simulink model "section_6_2_second_group"  (R2020a)
settings: Solver=ode45  StartTime=0.0  StopTime=50  RelTol=1e-5  EnableMultiTasking=on
(part 4 of 4)

== matlab function section_6_2_second_group/FUZZY2/fuzzy_adaptive_law2 ==
  data: wdot output; x1 input; x2 input; x3 input; zz input; w input
function wdot   = fcn(x1,x2,x3,zz,w)
delta=0.01;
ux1=zeros(5,1);
ux2=zeros(5,1);
ux3=zeros(5,1);
%%x1 5条模糊规则

z=zeros(5,6);
for j=1:5
    z(j,1)=-2+j-delta;
end
for j=6:10
    z(j-5,2)=-2+(j-5)-delta;
end
for j=11:15
    z(j-10,3)=-2+(j-10)-delta;
end

h1=1;%%规则间距
if x1<=-2-delta
    ux1(1,1)=1;
end

if x1>=-2-delta&&x1<=-1-delta
    ux1(1,1)=0.5*sin(pi*(x1-(-2-delta))/h1+0.5*pi)+0.5;
end

if x1>=-2-delta&&x1<=0-delta
    ux1(2,1)=0.5*sin(pi*(x1-(-1-delta))/h1+0.5*pi)+0.5;
end

if x1>=-1-delta&&x1<=1-delta
    ux1(3,1)=0.5*sin(pi*(x1-(0-delta))/h1+0.5*pi)+0.5;
end

if x1>=0-delta&&x1<=2-delta
    ux1(4,1)=0.5*sin(pi*(x1-(1-delta))/h1+0.5*pi)+0.5;
end

if x1>=1-delta&&x1<=2-delta
    ux1(5,1)=0.5*sin(pi*(x1-(2-delta))/h1+0.5*pi)+0.5;
end

if x1>2-delta
    ux1(5,1)=1;
end


h2=1;%%规则间距
if x2<=-2-delta
    ux2(1,1)=1;
end

if x2>=-2-delta&&x2<=-1-delta
    ux2(1,1)=0.5*sin(pi*(x2-(-2-delta))/h2+0.5*pi)+0.5;
end

if x2>=-2-delta&&x2<=0-delta
    ux2(2,1)=0.5*sin(pi*(x2-(-1-delta))/h2+0.5*pi)+0.5;
end

if x2>=-1-delta&&x2<=1-delta
    ux2(3,1)=0.5*sin(pi*(x2-(0-delta))/h2+0.5*pi)+0.5;
end

if x2>=0-delta&&x2<=2-delta
    ux2(4,1)=0.5*sin(pi*(x2-(1-delta))/h2+0.5*pi)+0.5;
end

if x2>=1-delta&&x2<=2-delta
    ux2(5,1)=0.5*sin(pi*(x2-(2-delta))/h2+0.5*pi)+0.5;
end

if x2>2-delta
    ux2(5,1)=1;
end

h3=1;%%规则间距
if x3<=-2-delta
    ux3(1,1)=1;
end

if x3>=-2-delta&&x3<=-1-delta
    ux3(1,1)=0.5*sin(pi*(x3-(-2-delta))/h3+0.5*pi)+0.5;
end

if x3>=-2-delta&&x3<=0-delta
    ux3(2,1)=0.5*sin(pi*(x3-(-1-delta))/h3+0.5*pi)+0.5;
end

if x3>=-1-delta&&x3<=1-delta
    ux3(3,1)=0.5*sin(pi*(x3-(0-delta))/h3+0.5*pi)+0.5;
end

if x3>=0-delta&&x3<=2-delta
    ux3(4,1)=0.5*sin(pi*(x3-(1-delta))/h3+0.5*pi)+0.5;
end

if x3>=1-delta&&x3<=2-delta
    ux3(5,1)=0.5*sin(pi*(x3-(2-delta))/h3+0.5*pi)+0.5;
end

if x3>2-delta
    ux3(5,1)=1;
end


%中心平均解模糊
Basic=0;
for i1=1:5
    for i2=1:5
        for i3=1:5
            Basic=Basic+ux1(i1,1)*ux2(i2,1)*ux3(i3,1);  
        end
    end
end

beta=zeros(5,5,5);
for i1=1:5
    for i2=1:5
        for i3=1:5
            beta(i1,i2,i3)=ux1(i1,1)*ux2(i2,1)*ux3(i3,1)/Basic;
        end
    end
end

wdot=zeros(5,5,5);
for i1=1:5
    for i2=1:5
        for i3=1:5
            wdot(i1,i2,i3)=w*beta(i1,i2,i3)*zz*z(i3,1);
        end
    end
end

end

== matlab function section_6_2_second_group/FUZZY2/fuzzy_adaptive_law3 ==
  data: wdot output; x1 input; x2 input; x3 input; zz input; w input
function wdot   = fcn(x1,x2,x3,zz,w)
delta=0.01;
ux1=zeros(5,1);
ux2=zeros(5,1);
ux3=zeros(5,1);
%%x1 5条模糊规则

z=zeros(5,6);
for j=1:5
    z(j,1)=-2+j-delta;
end
for j=6:10
    z(j-5,2)=-2+(j-5)-delta;
end
for j=11:15
    z(j-10,3)=-2+(j-10)-delta;
end

h1=1;%%规则间距
if x1<=-2-delta
    ux1(1,1)=1;
end

if x1>=-2-delta&&x1<=-1-delta
    ux1(1,1)=0.5*sin(pi*(x1-(-2-delta))/h1+0.5*pi)+0.5;
end

if x1>=-2-delta&&x1<=0-delta
    ux1(2,1)=0.5*sin(pi*(x1-(-1-delta))/h1+0.5*pi)+0.5;
end

if x1>=-1-delta&&x1<=1-delta
    ux1(3,1)=0.5*sin(pi*(x1-(0-delta))/h1+0.5*pi)+0.5;
end

if x1>=0-delta&&x1<=2-delta
    ux1(4,1)=0.5*sin(pi*(x1-(1-delta))/h1+0.5*pi)+0.5;
end

if x1>=1-delta&&x1<=2-delta
    ux1(5,1)=0.5*sin(pi*(x1-(2-delta))/h1+0.5*pi)+0.5;
end

if x1>2-delta
    ux1(5,1)=1;
end


h2=1;%%规则间距
if x2<=-2-delta
    ux2(1,1)=1;
end

if x2>=-2-delta&&x2<=-1-delta
    ux2(1,1)=0.5*sin(pi*(x2-(-2-delta))/h2+0.5*pi)+0.5;
end

if x2>=-2-delta&&x2<=0-delta
    ux2(2,1)=0.5*sin(pi*(x2-(-1-delta))/h2+0.5*pi)+0.5;
end

if x2>=-1-delta&&x2<=1-delta
    ux2(3,1)=0.5*sin(pi*(x2-(0-delta))/h2+0.5*pi)+0.5;
end

if x2>=0-delta&&x2<=2-delta
    ux2(4,1)=0.5*sin(pi*(x2-(1-delta))/h2+0.5*pi)+0.5;
end

if x2>=1-delta&&x2<=2-delta
    ux2(5,1)=0.5*sin(pi*(x2-(2-delta))/h2+0.5*pi)+0.5;
end

if x2>2-delta
    ux2(5,1)=1;
end

h3=1;%%规则间距
if x3<=-2-delta
    ux3(1,1)=1;
end

if x3>=-2-delta&&x3<=-1-delta
    ux3(1,1)=0.5*sin(pi*(x3-(-2-delta))/h3+0.5*pi)+0.5;
end

if x3>=-2-delta&&x3<=0-delta
    ux3(2,1)=0.5*sin(pi*(x3-(-1-delta))/h3+0.5*pi)+0.5;
end

if x3>=-1-delta&&x3<=1-delta
    ux3(3,1)=0.5*sin(pi*(x3-(0-delta))/h3+0.5*pi)+0.5;
end

if x3>=0-delta&&x3<=2-delta
    ux3(4,1)=0.5*sin(pi*(x3-(1-delta))/h3+0.5*pi)+0.5;
end

if x3>=1-delta&&x3<=2-delta
    ux3(5,1)=0.5*sin(pi*(x3-(2-delta))/h3+0.5*pi)+0.5;
end

if x3>2-delta
    ux3(5,1)=1;
end


%中心平均解模糊
Basic=0;
for i1=1:5
    for i2=1:5
        for i3=1:5
            Basic=Basic+ux1(i1,1)*ux2(i2,1)*ux3(i3,1);  
        end
    end
end

beta=zeros(5,5,5);
for i1=1:5
    for i2=1:5
        for i3=1:5
            beta(i1,i2,i3)=ux1(i1,1)*ux2(i2,1)*ux3(i3,1)/Basic;
        end
    end
end

wdot=zeros(5,5,5);
for i1=1:5
    for i2=1:5
        for i3=1:5
            wdot(i1,i2,i3)=w*beta(i1,i2,i3)*zz*z(i3,1);
        end
    end
end

end

== matlab function section_6_2_second_group/FUZZY2/fuzzy_adaptive_law4 ==
  data: wdot output; x1 input; x2 input; x3 input; zz input; w input
function wdot   = fcn(x1,x2,x3,zz,w)
delta=0.01;
ux1=zeros(5,1);
ux2=zeros(5,1);
ux3=zeros(5,1);
%%x1 5条模糊规则

z=zeros(5,6);
for j=1:5
    z(j,1)=-2+j-delta;
end
for j=6:10
    z(j-5,2)=-2+(j-5)-delta;
end
for j=11:15
    z(j-10,3)=-2+(j-10)-delta;
end

h1=1;%%规则间距
if x1<=-2-delta
    ux1(1,1)=1;
end

if x1>=-2-delta&&x1<=-1-delta
    ux1(1,1)=0.5*sin(pi*(x1-(-2-delta))/h1+0.5*pi)+0.5;
end

if x1>=-2-delta&&x1<=0-delta
    ux1(2,1)=0.5*sin(pi*(x1-(-1-delta))/h1+0.5*pi)+0.5;
end

if x1>=-1-delta&&x1<=1-delta
    ux1(3,1)=0.5*sin(pi*(x1-(0-delta))/h1+0.5*pi)+0.5;
end

if x1>=0-delta&&x1<=2-delta
    ux1(4,1)=0.5*sin(pi*(x1-(1-delta))/h1+0.5*pi)+0.5;
end

if x1>=1-delta&&x1<=2-delta
    ux1(5,1)=0.5*sin(pi*(x1-(2-delta))/h1+0.5*pi)+0.5;
end

if x1>2-delta
    ux1(5,1)=1;
end


h2=1;%%规则间距
if x2<=-2-delta
    ux2(1,1)=1;
end

if x2>=-2-delta&&x2<=-1-delta
    ux2(1,1)=0.5*sin(pi*(x2-(-2-delta))/h2+0.5*pi)+0.5;
end

if x2>=-2-delta&&x2<=0-delta
    ux2(2,1)=0.5*sin(pi*(x2-(-1-delta))/h2+0.5*pi)+0.5;
end

if x2>=-1-delta&&x2<=1-delta
    ux2(3,1)=0.5*sin(pi*(x2-(0-delta))/h2+0.5*pi)+0.5;
end

if x2>=0-delta&&x2<=2-delta
    ux2(4,1)=0.5*sin(pi*(x2-(1-delta))/h2+0.5*pi)+0.5;
end

if x2>=1-delta&&x2<=2-delta
    ux2(5,1)=0.5*sin(pi*(x2-(2-delta))/h2+0.5*pi)+0.5;
end

if x2>2-delta
    ux2(5,1)=1;
end

h3=1;%%规则间距
if x3<=-2-delta
    ux3(1,1)=1;
end

if x3>=-2-delta&&x3<=-1-delta
    ux3(1,1)=0.5*sin(pi*(x3-(-2-delta))/h3+0.5*pi)+0.5;
end

if x3>=-2-delta&&x3<=0-delta
    ux3(2,1)=0.5*sin(pi*(x3-(-1-delta))/h3+0.5*pi)+0.5;
end

if x3>=-1-delta&&x3<=1-delta
    ux3(3,1)=0.5*sin(pi*(x3-(0-delta))/h3+0.5*pi)+0.5;
end

if x3>=0-delta&&x3<=2-delta
    ux3(4,1)=0.5*sin(pi*(x3-(1-delta))/h3+0.5*pi)+0.5;
end

if x3>=1-delta&&x3<=2-delta
    ux3(5,1)=0.5*sin(pi*(x3-(2-delta))/h3+0.5*pi)+0.5;
end

if x3>2-delta
    ux3(5,1)=1;
end


%中心平均解模糊
Basic=0;
for i1=1:5
    for i2=1:5
        for i3=1:5
            Basic=Basic+ux1(i1,1)*ux2(i2,1)*ux3(i3,1);  
        end
    end
end

beta=zeros(5,5,5);
for i1=1:5
    for i2=1:5
        for i3=1:5
            beta(i1,i2,i3)=ux1(i1,1)*ux2(i2,1)*ux3(i3,1)/Basic;
        end
    end
end

wdot=zeros(5,5,5);
for i1=1:5
    for i2=1:5
        for i3=1:5
            wdot(i1,i2,i3)=w*beta(i1,i2,i3)*zz*z(i3,1);
        end
    end
end

end

== matlab function section_6_2_second_group/FUZZY2/fuzzy_adaptive_law5 ==
  data: wdot output; x1 input; x2 input; x3 input; zz input; w input
function wdot   = fcn(x1,x2,x3,zz,w)
delta=0.01;
ux1=zeros(5,1);
ux2=zeros(5,1);
ux3=zeros(5,1);
%%x1 5条模糊规则

z=zeros(5,6);
for j=1:5
    z(j,1)=-2+j-delta;
end
for j=6:10
    z(j-5,2)=-2+(j-5)-delta;
end
for j=11:15
    z(j-10,3)=-2+(j-10)-delta;
end

h1=1;%%规则间距
if x1<=-2-delta
    ux1(1,1)=1;
end

if x1>=-2-delta&&x1<=-1-delta
    ux1(1,1)=0.5*sin(pi*(x1-(-2-delta))/h1+0.5*pi)+0.5;
end

if x1>=-2-delta&&x1<=0-delta
    ux1(2,1)=0.5*sin(pi*(x1-(-1-delta))/h1+0.5*pi)+0.5;
end

if x1>=-1-delta&&x1<=1-delta
    ux1(3,1)=0.5*sin(pi*(x1-(0-delta))/h1+0.5*pi)+0.5;
end

if x1>=0-delta&&x1<=2-delta
    ux1(4,1)=0.5*sin(pi*(x1-(1-delta))/h1+0.5*pi)+0.5;
end

if x1>=1-delta&&x1<=2-delta
    ux1(5,1)=0.5*sin(pi*(x1-(2-delta))/h1+0.5*pi)+0.5;
end

if x1>2-delta
    ux1(5,1)=1;
end


h2=1;%%规则间距
if x2<=-2-delta
    ux2(1,1)=1;
end

if x2>=-2-delta&&x2<=-1-delta
    ux2(1,1)=0.5*sin(pi*(x2-(-2-delta))/h2+0.5*pi)+0.5;
end

if x2>=-2-delta&&x2<=0-delta
    ux2(2,1)=0.5*sin(pi*(x2-(-1-delta))/h2+0.5*pi)+0.5;
end

if x2>=-1-delta&&x2<=1-delta
    ux2(3,1)=0.5*sin(pi*(x2-(0-delta))/h2+0.5*pi)+0.5;
end

if x2>=0-delta&&x2<=2-delta
    ux2(4,1)=0.5*sin(pi*(x2-(1-delta))/h2+0.5*pi)+0.5;
end

if x2>=1-delta&&x2<=2-delta
    ux2(5,1)=0.5*sin(pi*(x2-(2-delta))/h2+0.5*pi)+0.5;
end

if x2>2-delta
    ux2(5,1)=1;
end

h3=1;%%规则间距
if x3<=-2-delta
    ux3(1,1)=1;
end

if x3>=-2-delta&&x3<=-1-delta
    ux3(1,1)=0.5*sin(pi*(x3-(-2-delta))/h3+0.5*pi)+0.5;
end

if x3>=-2-delta&&x3<=0-delta
    ux3(2,1)=0.5*sin(pi*(x3-(-1-delta))/h3+0.5*pi)+0.5;
end

if x3>=-1-delta&&x3<=1-delta
    ux3(3,1)=0.5*sin(pi*(x3-(0-delta))/h3+0.5*pi)+0.5;
end

if x3>=0-delta&&x3<=2-delta
    ux3(4,1)=0.5*sin(pi*(x3-(1-delta))/h3+0.5*pi)+0.5;
end

if x3>=1-delta&&x3<=2-delta
    ux3(5,1)=0.5*sin(pi*(x3-(2-delta))/h3+0.5*pi)+0.5;
end

if x3>2-delta
    ux3(5,1)=1;
end


%中心平均解模糊
Basic=0;
for i1=1:5
    for i2=1:5
        for i3=1:5
            Basic=Basic+ux1(i1,1)*ux2(i2,1)*ux3(i3,1);  
        end
    end
end

beta=zeros(5,5,5);
for i1=1:5
    for i2=1:5
        for i3=1:5
            beta(i1,i2,i3)=ux1(i1,1)*ux2(i2,1)*ux3(i3,1)/Basic;
        end
    end
end

wdot=zeros(5,5,5);
for i1=1:5
    for i2=1:5
        for i3=1:5
            wdot(i1,i2,i3)=w*beta(i1,i2,i3)*zz*z(i3,1);
        end
    end
end

end

== matlab function section_6_2_second_group/FUZZY2/fuzzy_adaptive_law6 ==
  data: wdot output; x1 input; x2 input; x3 input; zz input; w input
function wdot   = fcn(x1,x2,x3,zz,w)
delta=0.01;
ux1=zeros(5,1);
ux2=zeros(5,1);
ux3=zeros(5,1);
%%x1 5条模糊规则

z=zeros(5,6);
for j=1:5
    z(j,1)=-2+j-delta;
end
for j=6:10
    z(j-5,2)=-2+(j-5)-delta;
end
for j=11:15
    z(j-10,3)=-2+(j-10)-delta;
end

h1=1;%%规则间距
if x1<=-2-delta
    ux1(1,1)=1;
end

if x1>=-2-delta&&x1<=-1-delta
    ux1(1,1)=0.5*sin(pi*(x1-(-2-delta))/h1+0.5*pi)+0.5;
end

if x1>=-2-delta&&x1<=0-delta
    ux1(2,1)=0.5*sin(pi*(x1-(-1-delta))/h1+0.5*pi)+0.5;
end

if x1>=-1-delta&&x1<=1-delta
    ux1(3,1)=0.5*sin(pi*(x1-(0-delta))/h1+0.5*pi)+0.5;
end

if x1>=0-delta&&x1<=2-delta
    ux1(4,1)=0.5*sin(pi*(x1-(1-delta))/h1+0.5*pi)+0.5;
end

if x1>=1-delta&&x1<=2-delta
    ux1(5,1)=0.5*sin(pi*(x1-(2-delta))/h1+0.5*pi)+0.5;
end

if x1>2-delta
    ux1(5,1)=1;
end


h2=1;%%规则间距
if x2<=-2-delta
    ux2(1,1)=1;
end

if x2>=-2-delta&&x2<=-1-delta
    ux2(1,1)=0.5*sin(pi*(x2-(-2-delta))/h2+0.5*pi)+0.5;
end

if x2>=-2-delta&&x2<=0-delta
    ux2(2,1)=0.5*sin(pi*(x2-(-1-delta))/h2+0.5*pi)+0.5;
end

if x2>=-1-delta&&x2<=1-delta
    ux2(3,1)=0.5*sin(pi*(x2-(0-delta))/h2+0.5*pi)+0.5;
end

if x2>=0-delta&&x2<=2-delta
    ux2(4,1)=0.5*sin(pi*(x2-(1-delta))/h2+0.5*pi)+0.5;
end

if x2>=1-delta&&x2<=2-delta
    ux2(5,1)=0.5*sin(pi*(x2-(2-delta))/h2+0.5*pi)+0.5;
end

if x2>2-delta
    ux2(5,1)=1;
end

h3=1;%%规则间距
if x3<=-2-delta
    ux3(1,1)=1;
end

if x3>=-2-delta&&x3<=-1-delta
    ux3(1,1)=0.5*sin(pi*(x3-(-2-delta))/h3+0.5*pi)+0.5;
end

if x3>=-2-delta&&x3<=0-delta
    ux3(2,1)=0.5*sin(pi*(x3-(-1-delta))/h3+0.5*pi)+0.5;
end

if x3>=-1-delta&&x3<=1-delta
    ux3(3,1)=0.5*sin(pi*(x3-(0-delta))/h3+0.5*pi)+0.5;
end

if x3>=0-delta&&x3<=2-delta
    ux3(4,1)=0.5*sin(pi*(x3-(1-delta))/h3+0.5*pi)+0.5;
end

if x3>=1-delta&&x3<=2-delta
    ux3(5,1)=0.5*sin(pi*(x3-(2-delta))/h3+0.5*pi)+0.5;
end

if x3>2-delta
    ux3(5,1)=1;
end


%中心平均解模糊
Basic=0;
for i1=1:5
    for i2=1:5
        for i3=1:5
            Basic=Basic+ux1(i1,1)*ux2(i2,1)*ux3(i3,1);  
        end
    end
end

beta=zeros(5,5,5);
for i1=1:5
    for i2=1:5
        for i3=1:5
            beta(i1,i2,i3)=ux1(i1,1)*ux2(i2,1)*ux3(i3,1)/Basic;
        end
    end
end

wdot=zeros(5,5,5);
for i1=1:5
    for i2=1:5
        for i3=1:5
            wdot(i1,i2,i3)=w*beta(i1,i2,i3)*zz*z(i3,1);
        end
    end
end

end

== matlab function section_6_2_second_group/FUZZY2/fuzzy_adaptive_law7 ==
  data: wdot output; x1 input; x2 input; x3 input; zz input; w input
function wdot   = fcn(x1,x2,x3,zz,w)
delta=0.01;
ux1=zeros(5,1);
ux2=zeros(5,1);
ux3=zeros(5,1);
%%x1 5条模糊规则

z=zeros(5,6);
for j=1:5
    z(j,1)=-2+j-delta;
end
for j=6:10
    z(j-5,2)=-2+(j-5)-delta;
end
for j=11:15
    z(j-10,3)=-2+(j-10)-delta;
end

h1=1;%%规则间距
if x1<=-2-delta
    ux1(1,1)=1;
end

if x1>=-2-delta&&x1<=-1-delta
    ux1(1,1)=0.5*sin(pi*(x1-(-2-delta))/h1+0.5*pi)+0.5;
end

if x1>=-2-delta&&x1<=0-delta
    ux1(2,1)=0.5*sin(pi*(x1-(-1-delta))/h1+0.5*pi)+0.5;
end

if x1>=-1-delta&&x1<=1-delta
    ux1(3,1)=0.5*sin(pi*(x1-(0-delta))/h1+0.5*pi)+0.5;
end

if x1>=0-delta&&x1<=2-delta
    ux1(4,1)=0.5*sin(pi*(x1-(1-delta))/h1+0.5*pi)+0.5;
end

if x1>=1-delta&&x1<=2-delta
    ux1(5,1)=0.5*sin(pi*(x1-(2-delta))/h1+0.5*pi)+0.5;
end

if x1>2-delta
    ux1(5,1)=1;
end


h2=1;%%规则间距
if x2<=-2-delta
    ux2(1,1)=1;
end

if x2>=-2-delta&&x2<=-1-delta
    ux2(1,1)=0.5*sin(pi*(x2-(-2-delta))/h2+0.5*pi)+0.5;
end

if x2>=-2-delta&&x2<=0-delta
    ux2(2,1)=0.5*sin(pi*(x2-(-1-delta))/h2+0.5*pi)+0.5;
end

if x2>=-1-delta&&x2<=1-delta
    ux2(3,1)=0.5*sin(pi*(x2-(0-delta))/h2+0.5*pi)+0.5;
end

if x2>=0-delta&&x2<=2-delta
    ux2(4,1)=0.5*sin(pi*(x2-(1-delta))/h2+0.5*pi)+0.5;
end

if x2>=1-delta&&x2<=2-delta
    ux2(5,1)=0.5*sin(pi*(x2-(2-delta))/h2+0.5*pi)+0.5;
end

if x2>2-delta
    ux2(5,1)=1;
end

h3=1;%%规则间距
if x3<=-2-delta
    ux3(1,1)=1;
end

if x3>=-2-delta&&x3<=-1-delta
    ux3(1,1)=0.5*sin(pi*(x3-(-2-delta))/h3+0.5*pi)+0.5;
end

if x3>=-2-delta&&x3<=0-delta
    ux3(2,1)=0.5*sin(pi*(x3-(-1-delta))/h3+0.5*pi)+0.5;
end

if x3>=-1-delta&&x3<=1-delta
    ux3(3,1)=0.5*sin(pi*(x3-(0-delta))/h3+0.5*pi)+0.5;
end

if x3>=0-delta&&x3<=2-delta
    ux3(4,1)=0.5*sin(pi*(x3-(1-delta))/h3+0.5*pi)+0.5;
end

if x3>=1-delta&&x3<=2-delta
    ux3(5,1)=0.5*sin(pi*(x3-(2-delta))/h3+0.5*pi)+0.5;
end

if x3>2-delta
    ux3(5,1)=1;
end


%中心平均解模糊
Basic=0;
for i1=1:5
    for i2=1:5
        for i3=1:5
            Basic=Basic+ux1(i1,1)*ux2(i2,1)*ux3(i3,1);  
        end
    end
end

beta=zeros(5,5,5);
for i1=1:5
    for i2=1:5
        for i3=1:5
            beta(i1,i2,i3)=ux1(i1,1)*ux2(i2,1)*ux3(i3,1)/Basic;
        end
    end
end

wdot=zeros(5,5,5);
for i1=1:5
    for i2=1:5
        for i3=1:5
            wdot(i1,i2,i3)=w*beta(i1,i2,i3)*zz*z(i3,1);
        end
    end
end

end

== matlab function section_6_2_second_group/FUZZY2/fuzzy_adaptive_law8 ==
  data: wdot output; x1 input; x2 input; x3 input; zz input; w input
function wdot   = fcn(x1,x2,x3,zz,w)
delta=0.01;
ux1=zeros(5,1);
ux2=zeros(5,1);
ux3=zeros(5,1);
%%x1 5条模糊规则

z=zeros(5,6);
for j=1:5
    z(j,1)=-2+j-delta;
end
for j=6:10
    z(j-5,2)=-2+(j-5)-delta;
end
for j=11:15
    z(j-10,3)=-2+(j-10)-delta;
end

h1=1;%%规则间距
if x1<=-2-delta
    ux1(1,1)=1;
end

if x1>=-2-delta&&x1<=-1-delta
    ux1(1,1)=0.5*sin(pi*(x1-(-2-delta))/h1+0.5*pi)+0.5;
end

if x1>=-2-delta&&x1<=0-delta
    ux1(2,1)=0.5*sin(pi*(x1-(-1-delta))/h1+0.5*pi)+0.5;
end

if x1>=-1-delta&&x1<=1-delta
    ux1(3,1)=0.5*sin(pi*(x1-(0-delta))/h1+0.5*pi)+0.5;
end

if x1>=0-delta&&x1<=2-delta
    ux1(4,1)=0.5*sin(pi*(x1-(1-delta))/h1+0.5*pi)+0.5;
end

if x1>=1-delta&&x1<=2-delta
    ux1(5,1)=0.5*sin(pi*(x1-(2-delta))/h1+0.5*pi)+0.5;
end

if x1>2-delta
    ux1(5,1)=1;
end


h2=1;%%规则间距
if x2<=-2-delta
    ux2(1,1)=1;
end

if x2>=-2-delta&&x2<=-1-delta
    ux2(1,1)=0.5*sin(pi*(x2-(-2-delta))/h2+0.5*pi)+0.5;
end

if x2>=-2-delta&&x2<=0-delta
    ux2(2,1)=0.5*sin(pi*(x2-(-1-delta))/h2+0.5*pi)+0.5;
end

if x2>=-1-delta&&x2<=1-delta
    ux2(3,1)=0.5*sin(pi*(x2-(0-delta))/h2+0.5*pi)+0.5;
end

if x2>=0-delta&&x2<=2-delta
    ux2(4,1)=0.5*sin(pi*(x2-(1-delta))/h2+0.5*pi)+0.5;
end

if x2>=1-delta&&x2<=2-delta
    ux2(5,1)=0.5*sin(pi*(x2-(2-delta))/h2+0.5*pi)+0.5;
end

if x2>2-delta
    ux2(5,1)=1;
end

h3=1;%%规则间距
if x3<=-2-delta
    ux3(1,1)=1;
end

if x3>=-2-delta&&x3<=-1-delta
    ux3(1,1)=0.5*sin(pi*(x3-(-2-delta))/h3+0.5*pi)+0.5;
end

if x3>=-2-delta&&x3<=0-delta
    ux3(2,1)=0.5*sin(pi*(x3-(-1-delta))/h3+0.5*pi)+0.5;
end

if x3>=-1-delta&&x3<=1-delta
    ux3(3,1)=0.5*sin(pi*(x3-(0-delta))/h3+0.5*pi)+0.5;
end

if x3>=0-delta&&x3<=2-delta
    ux3(4,1)=0.5*sin(pi*(x3-(1-delta))/h3+0.5*pi)+0.5;
end

if x3>=1-delta&&x3<=2-delta
    ux3(5,1)=0.5*sin(pi*(x3-(2-delta))/h3+0.5*pi)+0.5;
end

if x3>2-delta
    ux3(5,1)=1;
end


%中心平均解模糊
Basic=0;
for i1=1:5
    for i2=1:5
        for i3=1:5
            Basic=Basic+ux1(i1,1)*ux2(i2,1)*ux3(i3,1);  
        end
    end
end

beta=zeros(5,5,5);
for i1=1:5
    for i2=1:5
        for i3=1:5
            beta(i1,i2,i3)=ux1(i1,1)*ux2(i2,1)*ux3(i3,1)/Basic;
        end
    end
end

wdot=zeros(5,5,5);
for i1=1:5
    for i2=1:5
        for i3=1:5
            wdot(i1,i2,i3)=w*beta(i1,i2,i3)*zz*z(i3,1);
        end
    end
end

end

== matlab function section_6_2_second_group/FUZZY2/fuzzy_adaptive_law9 ==
  data: wdot output; x1 input; x2 input; x3 input; zz input; w input
function wdot   = fcn(x1,x2,x3,zz,w)
delta=0.01;
ux1=zeros(5,1);
ux2=zeros(5,1);
ux3=zeros(5,1);
%%x1 5条模糊规则

z=zeros(5,6);
for j=1:5
    z(j,1)=-2+j-delta;
end
for j=6:10
    z(j-5,2)=-2+(j-5)-delta;
end
for j=11:15
    z(j-10,3)=-2+(j-10)-delta;
end

h1=1;%%规则间距
if x1<=-2-delta
    ux1(1,1)=1;
end

if x1>=-2-delta&&x1<=-1-delta
    ux1(1,1)=0.5*sin(pi*(x1-(-2-delta))/h1+0.5*pi)+0.5;
end

if x1>=-2-delta&&x1<=0-delta
    ux1(2,1)=0.5*sin(pi*(x1-(-1-delta))/h1+0.5*pi)+0.5;
end

if x1>=-1-delta&&x1<=1-delta
    ux1(3,1)=0.5*sin(pi*(x1-(0-delta))/h1+0.5*pi)+0.5;
end

if x1>=0-delta&&x1<=2-delta
    ux1(4,1)=0.5*sin(pi*(x1-(1-delta))/h1+0.5*pi)+0.5;
end

if x1>=1-delta&&x1<=2-delta
    ux1(5,1)=0.5*sin(pi*(x1-(2-delta))/h1+0.5*pi)+0.5;
end

if x1>2-delta
    ux1(5,1)=1;
end


h2=1;%%规则间距
if x2<=-2-delta
    ux2(1,1)=1;
end

if x2>=-2-delta&&x2<=-1-delta
    ux2(1,1)=0.5*sin(pi*(x2-(-2-delta))/h2+0.5*pi)+0.5;
end

if x2>=-2-delta&&x2<=0-delta
    ux2(2,1)=0.5*sin(pi*(x2-(-1-delta))/h2+0.5*pi)+0.5;
end

if x2>=-1-delta&&x2<=1-delta
    ux2(3,1)=0.5*sin(pi*(x2-(0-delta))/h2+0.5*pi)+0.5;
end

if x2>=0-delta&&x2<=2-delta
    ux2(4,1)=0.5*sin(pi*(x2-(1-delta))/h2+0.5*pi)+0.5;
end

if x2>=1-delta&&x2<=2-delta
    ux2(5,1)=0.5*sin(pi*(x2-(2-delta))/h2+0.5*pi)+0.5;
end

if x2>2-delta
    ux2(5,1)=1;
end

h3=1;%%规则间距
if x3<=-2-delta
    ux3(1,1)=1;
end

if x3>=-2-delta&&x3<=-1-delta
    ux3(1,1)=0.5*sin(pi*(x3-(-2-delta))/h3+0.5*pi)+0.5;
end

if x3>=-2-delta&&x3<=0-delta
    ux3(2,1)=0.5*sin(pi*(x3-(-1-delta))/h3+0.5*pi)+0.5;
end

if x3>=-1-delta&&x3<=1-delta
    ux3(3,1)=0.5*sin(pi*(x3-(0-delta))/h3+0.5*pi)+0.5;
end

if x3>=0-delta&&x3<=2-delta
    ux3(4,1)=0.5*sin(pi*(x3-(1-delta))/h3+0.5*pi)+0.5;
end

if x3>=1-delta&&x3<=2-delta
    ux3(5,1)=0.5*sin(pi*(x3-(2-delta))/h3+0.5*pi)+0.5;
end

if x3>2-delta
    ux3(5,1)=1;
end


%中心平均解模糊
Basic=0;
for i1=1:5
    for i2=1:5
        for i3=1:5
            Basic=Basic+ux1(i1,1)*ux2(i2,1)*ux3(i3,1);  
        end
    end
end

beta=zeros(5,5,5);
for i1=1:5
    for i2=1:5
        for i3=1:5
            beta(i1,i2,i3)=ux1(i1,1)*ux2(i2,1)*ux3(i3,1)/Basic;
        end
    end
end

wdot=zeros(5,5,5);
for i1=1:5
    for i2=1:5
        for i3=1:5
            wdot(i1,i2,i3)=w*beta(i1,i2,i3)*zz*z(i3,1);
        end
    end
end

end

== matlab function section_6_2_second_group/FUZZY2/fuzzy_logic_system1 ==
  data: aF output; x1 input; x2 input; x3 input; w input
function aF    = fcn(x1,x2,x3,w)
%%x1 5条模糊规则
delta=0.01;
ux1=zeros(5,1);
ux2=zeros(5,1);
ux3=zeros(5,1);
%%x1 5条模糊规则

h1=1;%%规则间距
if x1<=-2-delta
    ux1(1,1)=1;
end

if x1>=-2-delta&&x1<=-1-delta
    ux1(1,1)=0.5*sin(pi*(x1-(-2-delta))/h1+0.5*pi)+0.5;
end

if x1>=-2-delta&&x1<=0-delta
    ux1(2,1)=0.5*sin(pi*(x1-(-1-delta))/h1+0.5*pi)+0.5;
end

if x1>=-1-delta&&x1<=1-delta
    ux1(3,1)=0.5*sin(pi*(x1-(0-delta))/h1+0.5*pi)+0.5;
end

if x1>=0-delta&&x1<=2-delta
    ux1(4,1)=0.5*sin(pi*(x1-(1-delta))/h1+0.5*pi)+0.5;
end

if x1>=1-delta&&x1<=2-delta
    ux1(5,1)=0.5*sin(pi*(x1-(2-delta))/h1+0.5*pi)+0.5;
end

if x1>2-delta
    ux1(5,1)=1;
end


h2=1;%%规则间距
if x2<=-2-delta
    ux2(1,1)=1;
end

if x2>=-2-delta&&x2<=-1-delta
    ux2(1,1)=0.5*sin(pi*(x2-(-2-delta))/h2+0.5*pi)+0.5;
end

if x2>=-2-delta&&x2<=0-delta
    ux2(2,1)=0.5*sin(pi*(x2-(-1-delta))/h2+0.5*pi)+0.5;
end

if x2>=-1-delta&&x2<=1-delta
    ux2(3,1)=0.5*sin(pi*(x2-(0-delta))/h2+0.5*pi)+0.5;
end

if x2>=0-delta&&x2<=2-delta
    ux2(4,1)=0.5*sin(pi*(x2-(1-delta))/h2+0.5*pi)+0.5;
end

if x2>=1-delta&&x2<=2-delta
    ux2(5,1)=0.5*sin(pi*(x2-(2-delta))/h2+0.5*pi)+0.5;
end

if x2>2-delta
    ux2(5,1)=1;
end

h3=1;%%规则间距
if x3<=-2-delta
    ux3(1,1)=1;
end

if x3>=-2-delta&&x3<=-1-delta
    ux3(1,1)=0.5*sin(pi*(x3-(-2-delta))/h3+0.5*pi)+0.5;
end

if x3>=-2-delta&&x3<=0-delta
    ux3(2,1)=0.5*sin(pi*(x3-(-1-delta))/h3+0.5*pi)+0.5;
end

if x3>=-1-delta&&x3<=1-delta
    ux3(3,1)=0.5*sin(pi*(x3-(0-delta))/h3+0.5*pi)+0.5;
end

if x3>=0-delta&&x3<=2-delta
    ux3(4,1)=0.5*sin(pi*(x3-(1-delta))/h3+0.5*pi)+0.5;
end

if x3>=1-delta&&x3<=2-delta
    ux3(5,1)=0.5*sin(pi*(x3-(2-delta))/h3+0.5*pi)+0.5;
end

if x3>2-delta
    ux3(5,1)=1;
end



%中心平均解模糊
Basic=0;
for i1=1:5
    for i2=1:5
        for i3=1:5
            Basic=Basic+ux1(i1,1)*ux2(i2,1)*ux3(i3,1);
        end
    end
end

beta=zeros(5,5,5);
for i1=1:5
    for i2=1:5
        for i3=1:5
            beta(i1,i2,i3)=ux1(i1,1)*ux2(i2,1)*ux3(i3,1)/Basic;
        end
    end
end


aF=0;
for i1=1:5
    for i2=1:5
        for i3=1:5
            aF=aF+w(i1,i2,i3)*beta(i1,i2,i3); 
        end
    end
end

end

== matlab function section_6_2_second_group/FUZZY2/fuzzy_logic_system10 ==
  data: aF output; x1 input; x2 input; x3 input; w input
function aF    = fcn(x1,x2,x3,w)
%%x1 5条模糊规则
delta=0.01;
ux1=zeros(5,1);
ux2=zeros(5,1);
ux3=zeros(5,1);
%%x1 5条模糊规则

h1=1;%%规则间距
if x1<=-2-delta
    ux1(1,1)=1;
end

if x1>=-2-delta&&x1<=-1-delta
    ux1(1,1)=0.5*sin(pi*(x1-(-2-delta))/h1+0.5*pi)+0.5;
end

if x1>=-2-delta&&x1<=0-delta
    ux1(2,1)=0.5*sin(pi*(x1-(-1-delta))/h1+0.5*pi)+0.5;
end

if x1>=-1-delta&&x1<=1-delta
    ux1(3,1)=0.5*sin(pi*(x1-(0-delta))/h1+0.5*pi)+0.5;
end

if x1>=0-delta&&x1<=2-delta
    ux1(4,1)=0.5*sin(pi*(x1-(1-delta))/h1+0.5*pi)+0.5;
end

if x1>=1-delta&&x1<=2-delta
    ux1(5,1)=0.5*sin(pi*(x1-(2-delta))/h1+0.5*pi)+0.5;
end

if x1>2-delta
    ux1(5,1)=1;
end


h2=1;%%规则间距
if x2<=-2-delta
    ux2(1,1)=1;
end

if x2>=-2-delta&&x2<=-1-delta
    ux2(1,1)=0.5*sin(pi*(x2-(-2-delta))/h2+0.5*pi)+0.5;
end

if x2>=-2-delta&&x2<=0-delta
    ux2(2,1)=0.5*sin(pi*(x2-(-1-delta))/h2+0.5*pi)+0.5;
end

if x2>=-1-delta&&x2<=1-delta
    ux2(3,1)=0.5*sin(pi*(x2-(0-delta))/h2+0.5*pi)+0.5;
end

if x2>=0-delta&&x2<=2-delta
    ux2(4,1)=0.5*sin(pi*(x2-(1-delta))/h2+0.5*pi)+0.5;
end

if x2>=1-delta&&x2<=2-delta
    ux2(5,1)=0.5*sin(pi*(x2-(2-delta))/h2+0.5*pi)+0.5;
end

if x2>2-delta
    ux2(5,1)=1;
end

h3=1;%%规则间距
if x3<=-2-delta
    ux3(1,1)=1;
end

if x3>=-2-delta&&x3<=-1-delta
    ux3(1,1)=0.5*sin(pi*(x3-(-2-delta))/h3+0.5*pi)+0.5;
end

if x3>=-2-delta&&x3<=0-delta
    ux3(2,1)=0.5*sin(pi*(x3-(-1-delta))/h3+0.5*pi)+0.5;
end

if x3>=-1-delta&&x3<=1-delta
    ux3(3,1)=0.5*sin(pi*(x3-(0-delta))/h3+0.5*pi)+0.5;
end

if x3>=0-delta&&x3<=2-delta
    ux3(4,1)=0.5*sin(pi*(x3-(1-delta))/h3+0.5*pi)+0.5;
end

if x3>=1-delta&&x3<=2-delta
    ux3(5,1)=0.5*sin(pi*(x3-(2-delta))/h3+0.5*pi)+0.5;
end

if x3>2-delta
    ux3(5,1)=1;
end



%中心平均解模糊
Basic=0;
for i1=1:5
    for i2=1:5
        for i3=1:5
            Basic=Basic+ux1(i1,1)*ux2(i2,1)*ux3(i3,1);
        end
    end
end

beta=zeros(5,5,5);
for i1=1:5
    for i2=1:5
        for i3=1:5
            beta(i1,i2,i3)=ux1(i1,1)*ux2(i2,1)*ux3(i3,1)/Basic;
        end
    end
end


aF=0;
for i1=1:5
    for i2=1:5
        for i3=1:5
            aF=aF+w(i1,i2,i3)*beta(i1,i2,i3); 
        end
    end
end

end

== matlab function section_6_2_second_group/FUZZY2/fuzzy_logic_system2 ==
  data: aF output; x1 input; x2 input; x3 input; w input
function aF    = fcn(x1,x2,x3,w)
%%x1 5条模糊规则
delta=0.01;
ux1=zeros(5,1);
ux2=zeros(5,1);
ux3=zeros(5,1);
%%x1 5条模糊规则

h1=1;%%规则间距
if x1<=-2-delta
    ux1(1,1)=1;
end

if x1>=-2-delta&&x1<=-1-delta
    ux1(1,1)=0.5*sin(pi*(x1-(-2-delta))/h1+0.5*pi)+0.5;
end

if x1>=-2-delta&&x1<=0-delta
    ux1(2,1)=0.5*sin(pi*(x1-(-1-delta))/h1+0.5*pi)+0.5;
end

if x1>=-1-delta&&x1<=1-delta
    ux1(3,1)=0.5*sin(pi*(x1-(0-delta))/h1+0.5*pi)+0.5;
end

if x1>=0-delta&&x1<=2-delta
    ux1(4,1)=0.5*sin(pi*(x1-(1-delta))/h1+0.5*pi)+0.5;
end

if x1>=1-delta&&x1<=2-delta
    ux1(5,1)=0.5*sin(pi*(x1-(2-delta))/h1+0.5*pi)+0.5;
end

if x1>2-delta
    ux1(5,1)=1;
end


h2=1;%%规则间距
if x2<=-2-delta
    ux2(1,1)=1;
end

if x2>=-2-delta&&x2<=-1-delta
    ux2(1,1)=0.5*sin(pi*(x2-(-2-delta))/h2+0.5*pi)+0.5;
end

if x2>=-2-delta&&x2<=0-delta
    ux2(2,1)=0.5*sin(pi*(x2-(-1-delta))/h2+0.5*pi)+0.5;
end

if x2>=-1-delta&&x2<=1-delta
    ux2(3,1)=0.5*sin(pi*(x2-(0-delta))/h2+0.5*pi)+0.5;
end

if x2>=0-delta&&x2<=2-delta
    ux2(4,1)=0.5*sin(pi*(x2-(1-delta))/h2+0.5*pi)+0.5;
end

if x2>=1-delta&&x2<=2-delta
    ux2(5,1)=0.5*sin(pi*(x2-(2-delta))/h2+0.5*pi)+0.5;
end

if x2>2-delta
    ux2(5,1)=1;
end

h3=1;%%规则间距
if x3<=-2-delta
    ux3(1,1)=1;
end

if x3>=-2-delta&&x3<=-1-delta
    ux3(1,1)=0.5*sin(pi*(x3-(-2-delta))/h3+0.5*pi)+0.5;
end

if x3>=-2-delta&&x3<=0-delta
    ux3(2,1)=0.5*sin(pi*(x3-(-1-delta))/h3+0.5*pi)+0.5;
end

if x3>=-1-delta&&x3<=1-delta
    ux3(3,1)=0.5*sin(pi*(x3-(0-delta))/h3+0.5*pi)+0.5;
end

if x3>=0-delta&&x3<=2-delta
    ux3(4,1)=0.5*sin(pi*(x3-(1-delta))/h3+0.5*pi)+0.5;
end

if x3>=1-delta&&x3<=2-delta
    ux3(5,1)=0.5*sin(pi*(x3-(2-delta))/h3+0.5*pi)+0.5;
end

if x3>2-delta
    ux3(5,1)=1;
end



%中心平均解模糊
Basic=0;
for i1=1:5
    for i2=1:5
        for i3=1:5
            Basic=Basic+ux1(i1,1)*ux2(i2,1)*ux3(i3,1);
        end
    end
end

beta=zeros(5,5,5);
for i1=1:5
    for i2=1:5
        for i3=1:5
            beta(i1,i2,i3)=ux1(i1,1)*ux2(i2,1)*ux3(i3,1)/Basic;
        end
    end
end


aF=0;
for i1=1:5
    for i2=1:5
        for i3=1:5
            aF=aF+w(i1,i2,i3)*beta(i1,i2,i3); 
        end
    end
end

end

== matlab function section_6_2_second_group/FUZZY2/fuzzy_logic_system3 ==
  data: aF output; x1 input; x2 input; x3 input; w input
function aF    = fcn(x1,x2,x3,w)
%%x1 5条模糊规则
delta=0.01;
ux1=zeros(5,1);
ux2=zeros(5,1);
ux3=zeros(5,1);
%%x1 5条模糊规则

h1=1;%%规则间距
if x1<=-2-delta
    ux1(1,1)=1;
end

if x1>=-2-delta&&x1<=-1-delta
    ux1(1,1)=0.5*sin(pi*(x1-(-2-delta))/h1+0.5*pi)+0.5;
end

if x1>=-2-delta&&x1<=0-delta
    ux1(2,1)=0.5*sin(pi*(x1-(-1-delta))/h1+0.5*pi)+0.5;
end

if x1>=-1-delta&&x1<=1-delta
    ux1(3,1)=0.5*sin(pi*(x1-(0-delta))/h1+0.5*pi)+0.5;
end

if x1>=0-delta&&x1<=2-delta
    ux1(4,1)=0.5*sin(pi*(x1-(1-delta))/h1+0.5*pi)+0.5;
end

if x1>=1-delta&&x1<=2-delta
    ux1(5,1)=0.5*sin(pi*(x1-(2-delta))/h1+0.5*pi)+0.5;
end

if x1>2-delta
    ux1(5,1)=1;
end


h2=1;%%规则间距
if x2<=-2-delta
    ux2(1,1)=1;
end

if x2>=-2-delta&&x2<=-1-delta
    ux2(1,1)=0.5*sin(pi*(x2-(-2-delta))/h2+0.5*pi)+0.5;
end

if x2>=-2-delta&&x2<=0-delta
    ux2(2,1)=0.5*sin(pi*(x2-(-1-delta))/h2+0.5*pi)+0.5;
end

if x2>=-1-delta&&x2<=1-delta
    ux2(3,1)=0.5*sin(pi*(x2-(0-delta))/h2+0.5*pi)+0.5;
end

if x2>=0-delta&&x2<=2-delta
    ux2(4,1)=0.5*sin(pi*(x2-(1-delta))/h2+0.5*pi)+0.5;
end

if x2>=1-delta&&x2<=2-delta
    ux2(5,1)=0.5*sin(pi*(x2-(2-delta))/h2+0.5*pi)+0.5;
end

if x2>2-delta
    ux2(5,1)=1;
end

h3=1;%%规则间距
if x3<=-2-delta
    ux3(1,1)=1;
end

if x3>=-2-delta&&x3<=-1-delta
    ux3(1,1)=0.5*sin(pi*(x3-(-2-delta))/h3+0.5*pi)+0.5;
end

if x3>=-2-delta&&x3<=0-delta
    ux3(2,1)=0.5*sin(pi*(x3-(-1-delta))/h3+0.5*pi)+0.5;
end

if x3>=-1-delta&&x3<=1-delta
    ux3(3,1)=0.5*sin(pi*(x3-(0-delta))/h3+0.5*pi)+0.5;
end

if x3>=0-delta&&x3<=2-delta
    ux3(4,1)=0.5*sin(pi*(x3-(1-delta))/h3+0.5*pi)+0.5;
end

if x3>=1-delta&&x3<=2-delta
    ux3(5,1)=0.5*sin(pi*(x3-(2-delta))/h3+0.5*pi)+0.5;
end

if x3>2-delta
    ux3(5,1)=1;
end



%中心平均解模糊
Basic=0;
for i1=1:5
    for i2=1:5
        for i3=1:5
            Basic=Basic+ux1(i1,1)*ux2(i2,1)*ux3(i3,1);
        end
    end
end

beta=zeros(5,5,5);
for i1=1:5
    for i2=1:5
        for i3=1:5
            beta(i1,i2,i3)=ux1(i1,1)*ux2(i2,1)*ux3(i3,1)/Basic;
        end
    end
end


aF=0;
for i1=1:5
    for i2=1:5
        for i3=1:5
            aF=aF+w(i1,i2,i3)*beta(i1,i2,i3); 
        end
    end
end

end

== matlab function section_6_2_second_group/FUZZY2/fuzzy_logic_system4 ==
  data: aF output; x1 input; x2 input; x3 input; w input
function aF    = fcn(x1,x2,x3,w)
%%x1 5条模糊规则
delta=0.01;
ux1=zeros(5,1);
ux2=zeros(5,1);
ux3=zeros(5,1);
%%x1 5条模糊规则

h1=1;%%规则间距
if x1<=-2-delta
    ux1(1,1)=1;
end

if x1>=-2-delta&&x1<=-1-delta
    ux1(1,1)=0.5*sin(pi*(x1-(-2-delta))/h1+0.5*pi)+0.5;
end

if x1>=-2-delta&&x1<=0-delta
    ux1(2,1)=0.5*sin(pi*(x1-(-1-delta))/h1+0.5*pi)+0.5;
end

if x1>=-1-delta&&x1<=1-delta
    ux1(3,1)=0.5*sin(pi*(x1-(0-delta))/h1+0.5*pi)+0.5;
end

if x1>=0-delta&&x1<=2-delta
    ux1(4,1)=0.5*sin(pi*(x1-(1-delta))/h1+0.5*pi)+0.5;
end

if x1>=1-delta&&x1<=2-delta
    ux1(5,1)=0.5*sin(pi*(x1-(2-delta))/h1+0.5*pi)+0.5;
end

if x1>2-delta
    ux1(5,1)=1;
end


h2=1;%%规则间距
if x2<=-2-delta
    ux2(1,1)=1;
end

if x2>=-2-delta&&x2<=-1-delta
    ux2(1,1)=0.5*sin(pi*(x2-(-2-delta))/h2+0.5*pi)+0.5;
end

if x2>=-2-delta&&x2<=0-delta
    ux2(2,1)=0.5*sin(pi*(x2-(-1-delta))/h2+0.5*pi)+0.5;
end

if x2>=-1-delta&&x2<=1-delta
    ux2(3,1)=0.5*sin(pi*(x2-(0-delta))/h2+0.5*pi)+0.5;
end

if x2>=0-delta&&x2<=2-delta
    ux2(4,1)=0.5*sin(pi*(x2-(1-delta))/h2+0.5*pi)+0.5;
end

if x2>=1-delta&&x2<=2-delta
    ux2(5,1)=0.5*sin(pi*(x2-(2-delta))/h2+0.5*pi)+0.5;
end

if x2>2-delta
    ux2(5,1)=1;
end

h3=1;%%规则间距
if x3<=-2-delta
    ux3(1,1)=1;
end

if x3>=-2-delta&&x3<=-1-delta
    ux3(1,1)=0.5*sin(pi*(x3-(-2-delta))/h3+0.5*pi)+0.5;
end

if x3>=-2-delta&&x3<=0-delta
    ux3(2,1)=0.5*sin(pi*(x3-(-1-delta))/h3+0.5*pi)+0.5;
end

if x3>=-1-delta&&x3<=1-delta
    ux3(3,1)=0.5*sin(pi*(x3-(0-delta))/h3+0.5*pi)+0.5;
end

if x3>=0-delta&&x3<=2-delta
    ux3(4,1)=0.5*sin(pi*(x3-(1-delta))/h3+0.5*pi)+0.5;
end

if x3>=1-delta&&x3<=2-delta
    ux3(5,1)=0.5*sin(pi*(x3-(2-delta))/h3+0.5*pi)+0.5;
end

if x3>2-delta
    ux3(5,1)=1;
end



%中心平均解模糊
Basic=0;
for i1=1:5
    for i2=1:5
        for i3=1:5
            Basic=Basic+ux1(i1,1)*ux2(i2,1)*ux3(i3,1);
        end
    end
end

beta=zeros(5,5,5);
for i1=1:5
    for i2=1:5
        for i3=1:5
            beta(i1,i2,i3)=ux1(i1,1)*ux2(i2,1)*ux3(i3,1)/Basic;
        end
    end
end


aF=0;
for i1=1:5
    for i2=1:5
        for i3=1:5
            aF=aF+w(i1,i2,i3)*beta(i1,i2,i3); 
        end
    end
end

end

== matlab function section_6_2_second_group/FUZZY2/fuzzy_logic_system5 ==
  data: aF output; x1 input; x2 input; x3 input; w input
function aF    = fcn(x1,x2,x3,w)
%%x1 5条模糊规则
delta=0.01;
ux1=zeros(5,1);
ux2=zeros(5,1);
ux3=zeros(5,1);
%%x1 5条模糊规则

h1=1;%%规则间距
if x1<=-2-delta
    ux1(1,1)=1;
end

if x1>=-2-delta&&x1<=-1-delta
    ux1(1,1)=0.5*sin(pi*(x1-(-2-delta))/h1+0.5*pi)+0.5;
end

if x1>=-2-delta&&x1<=0-delta
    ux1(2,1)=0.5*sin(pi*(x1-(-1-delta))/h1+0.5*pi)+0.5;
end

if x1>=-1-delta&&x1<=1-delta
    ux1(3,1)=0.5*sin(pi*(x1-(0-delta))/h1+0.5*pi)+0.5;
end

if x1>=0-delta&&x1<=2-delta
    ux1(4,1)=0.5*sin(pi*(x1-(1-delta))/h1+0.5*pi)+0.5;
end

if x1>=1-delta&&x1<=2-delta
    ux1(5,1)=0.5*sin(pi*(x1-(2-delta))/h1+0.5*pi)+0.5;
end

if x1>2-delta
    ux1(5,1)=1;
end


h2=1;%%规则间距
if x2<=-2-delta
    ux2(1,1)=1;
end

if x2>=-2-delta&&x2<=-1-delta
    ux2(1,1)=0.5*sin(pi*(x2-(-2-delta))/h2+0.5*pi)+0.5;
end

if x2>=-2-delta&&x2<=0-delta
    ux2(2,1)=0.5*sin(pi*(x2-(-1-delta))/h2+0.5*pi)+0.5;
end

if x2>=-1-delta&&x2<=1-delta
    ux2(3,1)=0.5*sin(pi*(x2-(0-delta))/h2+0.5*pi)+0.5;
end

if x2>=0-delta&&x2<=2-delta
    ux2(4,1)=0.5*sin(pi*(x2-(1-delta))/h2+0.5*pi)+0.5;
end

if x2>=1-delta&&x2<=2-delta
    ux2(5,1)=0.5*sin(pi*(x2-(2-delta))/h2+0.5*pi)+0.5;
end

if x2>2-delta
    ux2(5,1)=1;
end

h3=1;%%规则间距
if x3<=-2-delta
    ux3(1,1)=1;
end

if x3>=-2-delta&&x3<=-1-delta
    ux3(1,1)=0.5*sin(pi*(x3-(-2-delta))/h3+0.5*pi)+0.5;
end

if x3>=-2-delta&&x3<=0-delta
    ux3(2,1)=0.5*sin(pi*(x3-(-1-delta))/h3+0.5*pi)+0.5;
end

if x3>=-1-delta&&x3<=1-delta
    ux3(3,1)=0.5*sin(pi*(x3-(0-delta))/h3+0.5*pi)+0.5;
end

if x3>=0-delta&&x3<=2-delta
    ux3(4,1)=0.5*sin(pi*(x3-(1-delta))/h3+0.5*pi)+0.5;
end

if x3>=1-delta&&x3<=2-delta
    ux3(5,1)=0.5*sin(pi*(x3-(2-delta))/h3+0.5*pi)+0.5;
end

if x3>2-delta
    ux3(5,1)=1;
end



%中心平均解模糊
Basic=0;
for i1=1:5
    for i2=1:5
        for i3=1:5
            Basic=Basic+ux1(i1,1)*ux2(i2,1)*ux3(i3,1);
        end
    end
end

beta=zeros(5,5,5);
for i1=1:5
    for i2=1:5
        for i3=1:5
            beta(i1,i2,i3)=ux1(i1,1)*ux2(i2,1)*ux3(i3,1)/Basic;
        end
    end
end


aF=0;
for i1=1:5
    for i2=1:5
        for i3=1:5
            aF=aF+w(i1,i2,i3)*beta(i1,i2,i3); 
        end
    end
end

end

== matlab function section_6_2_second_group/FUZZY2/fuzzy_logic_system6 ==
  data: aF output; x1 input; x2 input; x3 input; w input
function aF    = fcn(x1,x2,x3,w)
%%x1 5条模糊规则
delta=0.01;
ux1=zeros(5,1);
ux2=zeros(5,1);
ux3=zeros(5,1);
%%x1 5条模糊规则

h1=1;%%规则间距
if x1<=-2-delta
    ux1(1,1)=1;
end

if x1>=-2-delta&&x1<=-1-delta
    ux1(1,1)=0.5*sin(pi*(x1-(-2-delta))/h1+0.5*pi)+0.5;
end

if x1>=-2-delta&&x1<=0-delta
    ux1(2,1)=0.5*sin(pi*(x1-(-1-delta))/h1+0.5*pi)+0.5;
end

if x1>=-1-delta&&x1<=1-delta
    ux1(3,1)=0.5*sin(pi*(x1-(0-delta))/h1+0.5*pi)+0.5;
end

if x1>=0-delta&&x1<=2-delta
    ux1(4,1)=0.5*sin(pi*(x1-(1-delta))/h1+0.5*pi)+0.5;
end

if x1>=1-delta&&x1<=2-delta
    ux1(5,1)=0.5*sin(pi*(x1-(2-delta))/h1+0.5*pi)+0.5;
end

if x1>2-delta
    ux1(5,1)=1;
end


h2=1;%%规则间距
if x2<=-2-delta
    ux2(1,1)=1;
end

if x2>=-2-delta&&x2<=-1-delta
    ux2(1,1)=0.5*sin(pi*(x2-(-2-delta))/h2+0.5*pi)+0.5;
end

if x2>=-2-delta&&x2<=0-delta
    ux2(2,1)=0.5*sin(pi*(x2-(-1-delta))/h2+0.5*pi)+0.5;
end

if x2>=-1-delta&&x2<=1-delta
    ux2(3,1)=0.5*sin(pi*(x2-(0-delta))/h2+0.5*pi)+0.5;
end

if x2>=0-delta&&x2<=2-delta
    ux2(4,1)=0.5*sin(pi*(x2-(1-delta))/h2+0.5*pi)+0.5;
end

if x2>=1-delta&&x2<=2-delta
    ux2(5,1)=0.5*sin(pi*(x2-(2-delta))/h2+0.5*pi)+0.5;
end

if x2>2-delta
    ux2(5,1)=1;
end

h3=1;%%规则间距
if x3<=-2-delta
    ux3(1,1)=1;
end

if x3>=-2-delta&&x3<=-1-delta
    ux3(1,1)=0.5*sin(pi*(x3-(-2-delta))/h3+0.5*pi)+0.5;
end

if x3>=-2-delta&&x3<=0-delta
    ux3(2,1)=0.5*sin(pi*(x3-(-1-delta))/h3+0.5*pi)+0.5;
end

if x3>=-1-delta&&x3<=1-delta
    ux3(3,1)=0.5*sin(pi*(x3-(0-delta))/h3+0.5*pi)+0.5;
end

if x3>=0-delta&&x3<=2-delta
    ux3(4,1)=0.5*sin(pi*(x3-(1-delta))/h3+0.5*pi)+0.5;
end

if x3>=1-delta&&x3<=2-delta
    ux3(5,1)=0.5*sin(pi*(x3-(2-delta))/h3+0.5*pi)+0.5;
end

if x3>2-delta
    ux3(5,1)=1;
end



%中心平均解模糊
Basic=0;
for i1=1:5
    for i2=1:5
        for i3=1:5
            Basic=Basic+ux1(i1,1)*ux2(i2,1)*ux3(i3,1);
        end
    end
end

beta=zeros(5,5,5);
for i1=1:5
    for i2=1:5
        for i3=1:5
            beta(i1,i2,i3)=ux1(i1,1)*ux2(i2,1)*ux3(i3,1)/Basic;
        end
    end
end


aF=0;
for i1=1:5
    for i2=1:5
        for i3=1:5
            aF=aF+w(i1,i2,i3)*beta(i1,i2,i3); 
        end
    end
end

end

== matlab function section_6_2_second_group/FUZZY2/fuzzy_logic_system7 ==
  data: aF output; x1 input; x2 input; x3 input; w input
function aF    = fcn(x1,x2,x3,w)
%%x1 5条模糊规则
delta=0.01;
ux1=zeros(5,1);
ux2=zeros(5,1);
ux3=zeros(5,1);
%%x1 5条模糊规则

h1=1;%%规则间距
if x1<=-2-delta
    ux1(1,1)=1;
end

if x1>=-2-delta&&x1<=-1-delta
    ux1(1,1)=0.5*sin(pi*(x1-(-2-delta))/h1+0.5*pi)+0.5;
end

if x1>=-2-delta&&x1<=0-delta
    ux1(2,1)=0.5*sin(pi*(x1-(-1-delta))/h1+0.5*pi)+0.5;
end

if x1>=-1-delta&&x1<=1-delta
    ux1(3,1)=0.5*sin(pi*(x1-(0-delta))/h1+0.5*pi)+0.5;
end

if x1>=0-delta&&x1<=2-delta
    ux1(4,1)=0.5*sin(pi*(x1-(1-delta))/h1+0.5*pi)+0.5;
end

if x1>=1-delta&&x1<=2-delta
    ux1(5,1)=0.5*sin(pi*(x1-(2-delta))/h1+0.5*pi)+0.5;
end

if x1>2-delta
    ux1(5,1)=1;
end


h2=1;%%规则间距
if x2<=-2-delta
    ux2(1,1)=1;
end

if x2>=-2-delta&&x2<=-1-delta
    ux2(1,1)=0.5*sin(pi*(x2-(-2-delta))/h2+0.5*pi)+0.5;
end

if x2>=-2-delta&&x2<=0-delta
    ux2(2,1)=0.5*sin(pi*(x2-(-1-delta))/h2+0.5*pi)+0.5;
end

if x2>=-1-delta&&x2<=1-delta
    ux2(3,1)=0.5*sin(pi*(x2-(0-delta))/h2+0.5*pi)+0.5;
end

if x2>=0-delta&&x2<=2-delta
    ux2(4,1)=0.5*sin(pi*(x2-(1-delta))/h2+0.5*pi)+0.5;
end

if x2>=1-delta&&x2<=2-delta
    ux2(5,1)=0.5*sin(pi*(x2-(2-delta))/h2+0.5*pi)+0.5;
end

if x2>2-delta
    ux2(5,1)=1;
end

h3=1;%%规则间距
if x3<=-2-delta
    ux3(1,1)=1;
end

if x3>=-2-delta&&x3<=-1-delta
    ux3(1,1)=0.5*sin(pi*(x3-(-2-delta))/h3+0.5*pi)+0.5;
end

if x3>=-2-delta&&x3<=0-delta
    ux3(2,1)=0.5*sin(pi*(x3-(-1-delta))/h3+0.5*pi)+0.5;
end

if x3>=-1-delta&&x3<=1-delta
    ux3(3,1)=0.5*sin(pi*(x3-(0-delta))/h3+0.5*pi)+0.5;
end

if x3>=0-delta&&x3<=2-delta
    ux3(4,1)=0.5*sin(pi*(x3-(1-delta))/h3+0.5*pi)+0.5;
end

if x3>=1-delta&&x3<=2-delta
    ux3(5,1)=0.5*sin(pi*(x3-(2-delta))/h3+0.5*pi)+0.5;
end

if x3>2-delta
    ux3(5,1)=1;
end



%中心平均解模糊
Basic=0;
for i1=1:5
    for i2=1:5
        for i3=1:5
            Basic=Basic+ux1(i1,1)*ux2(i2,1)*ux3(i3,1);
        end
    end
end

beta=zeros(5,5,5);
for i1=1:5
    for i2=1:5
        for i3=1:5
            beta(i1,i2,i3)=ux1(i1,1)*ux2(i2,1)*ux3(i3,1)/Basic;
        end
    end
end


aF=0;
for i1=1:5
    for i2=1:5
        for i3=1:5
            aF=aF+w(i1,i2,i3)*beta(i1,i2,i3); 
        end
    end
end

end

== matlab function section_6_2_second_group/FUZZY2/fuzzy_logic_system8 ==
  data: aF output; x1 input; x2 input; x3 input; w input
function aF    = fcn(x1,x2,x3,w)
%%x1 5条模糊规则
delta=0.01;
ux1=zeros(5,1);
ux2=zeros(5,1);
ux3=zeros(5,1);
%%x1 5条模糊规则

h1=1;%%规则间距
if x1<=-2-delta
    ux1(1,1)=1;
end

if x1>=-2-delta&&x1<=-1-delta
    ux1(1,1)=0.5*sin(pi*(x1-(-2-delta))/h1+0.5*pi)+0.5;
end

if x1>=-2-delta&&x1<=0-delta
    ux1(2,1)=0.5*sin(pi*(x1-(-1-delta))/h1+0.5*pi)+0.5;
end

if x1>=-1-delta&&x1<=1-delta
    ux1(3,1)=0.5*sin(pi*(x1-(0-delta))/h1+0.5*pi)+0.5;
end

if x1>=0-delta&&x1<=2-delta
    ux1(4,1)=0.5*sin(pi*(x1-(1-delta))/h1+0.5*pi)+0.5;
end

if x1>=1-delta&&x1<=2-delta
    ux1(5,1)=0.5*sin(pi*(x1-(2-delta))/h1+0.5*pi)+0.5;
end

if x1>2-delta
    ux1(5,1)=1;
end


h2=1;%%规则间距
if x2<=-2-delta
    ux2(1,1)=1;
end

if x2>=-2-delta&&x2<=-1-delta
    ux2(1,1)=0.5*sin(pi*(x2-(-2-delta))/h2+0.5*pi)+0.5;
end

if x2>=-2-delta&&x2<=0-delta
    ux2(2,1)=0.5*sin(pi*(x2-(-1-delta))/h2+0.5*pi)+0.5;
end

if x2>=-1-delta&&x2<=1-delta
    ux2(3,1)=0.5*sin(pi*(x2-(0-delta))/h2+0.5*pi)+0.5;
end

if x2>=0-delta&&x2<=2-delta
    ux2(4,1)=0.5*sin(pi*(x2-(1-delta))/h2+0.5*pi)+0.5;
end

if x2>=1-delta&&x2<=2-delta
    ux2(5,1)=0.5*sin(pi*(x2-(2-delta))/h2+0.5*pi)+0.5;
end

if x2>2-delta
    ux2(5,1)=1;
end

h3=1;%%规则间距
if x3<=-2-delta
    ux3(1,1)=1;
end

if x3>=-2-delta&&x3<=-1-delta
    ux3(1,1)=0.5*sin(pi*(x3-(-2-delta))/h3+0.5*pi)+0.5;
end

if x3>=-2-delta&&x3<=0-delta
    ux3(2,1)=0.5*sin(pi*(x3-(-1-delta))/h3+0.5*pi)+0.5;
end

if x3>=-1-delta&&x3<=1-delta
    ux3(3,1)=0.5*sin(pi*(x3-(0-delta))/h3+0.5*pi)+0.5;
end

if x3>=0-delta&&x3<=2-delta
    ux3(4,1)=0.5*sin(pi*(x3-(1-delta))/h3+0.5*pi)+0.5;
end

if x3>=1-delta&&x3<=2-delta
    ux3(5,1)=0.5*sin(pi*(x3-(2-delta))/h3+0.5*pi)+0.5;
end

if x3>2-delta
    ux3(5,1)=1;
end



%中心平均解模糊
Basic=0;
for i1=1:5
    for i2=1:5
        for i3=1:5
            Basic=Basic+ux1(i1,1)*ux2(i2,1)*ux3(i3,1);
        end
    end
end

beta=zeros(5,5,5);
for i1=1:5
    for i2=1:5
        for i3=1:5
            beta(i1,i2,i3)=ux1(i1,1)*ux2(i2,1)*ux3(i3,1)/Basic;
        end
    end
end


aF=0;
for i1=1:5
    for i2=1:5
        for i3=1:5
            aF=aF+w(i1,i2,i3)*beta(i1,i2,i3); 
        end
    end
end

end

== matlab function section_6_2_second_group/FUZZY3/2D-3D1 ==
  data: y output; x input
function y  = fcn(x)
y=zeros(5,5,5);

for i=1:5
    for j=1:5
        for k=1:5
            y(i,j,k)=x(5*(k-1)+i,j);
        end
    end
end

end

== matlab function section_6_2_second_group/FUZZY3/2D-3D2 ==
  data: y output; x input
function y  = fcn(x)
y=zeros(5,5,5);

for i=1:5
    for j=1:5
        for k=1:5
            y(i,j,k)=x(5*(k-1)+i,j);
        end
    end
end

end

== matlab function section_6_2_second_group/FUZZY3/2D-3D3 ==
  data: y output; x input
function y  = fcn(x)
y=zeros(5,5,5);

for i=1:5
    for j=1:5
        for k=1:5
            y(i,j,k)=x(5*(k-1)+i,j);
        end
    end
end

end

== matlab function section_6_2_second_group/FUZZY3/2D-3D4 ==
  data: y output; x input
function y  = fcn(x)
y=zeros(5,5,5);

for i=1:5
    for j=1:5
        for k=1:5
            y(i,j,k)=x(5*(k-1)+i,j);
        end
    end
end

end

== matlab function section_6_2_second_group/FUZZY3/2D-3D5 ==
  data: y output; x input
function y  = fcn(x)
y=zeros(5,5,5);

for i=1:5
    for j=1:5
        for k=1:5
            y(i,j,k)=x(5*(k-1)+i,j);
        end
    end
end

end

== matlab function section_6_2_second_group/FUZZY3/2D-3D6 ==
  data: y output; x input
function y  = fcn(x)
y=zeros(5,5,5);

for i=1:5
    for j=1:5
        for k=1:5
            y(i,j,k)=x(5*(k-1)+i,j);
        end
    end
end

end

== matlab function section_6_2_second_group/FUZZY3/2D-3D7 ==
  data: y output; x input
function y  = fcn(x)
y=zeros(5,5,5);

for i=1:5
    for j=1:5
        for k=1:5
            y(i,j,k)=x(5*(k-1)+i,j);
        end
    end
end

end

== matlab function section_6_2_second_group/FUZZY3/2D-3D8 ==
  data: y output; x input
function y  = fcn(x)
y=zeros(5,5,5);

for i=1:5
    for j=1:5
        for k=1:5
            y(i,j,k)=x(5*(k-1)+i,j);
        end
    end
end

end

== matlab function section_6_2_second_group/FUZZY3/2D-3D9 ==
  data: y output; x input
function y  = fcn(x)
y=zeros(5,5,5);

for i=1:5
    for j=1:5
        for k=1:5
            y(i,j,k)=x(5*(k-1)+i,j);
        end
    end
end

end

== matlab function section_6_2_second_group/FUZZY3/3D-2D1 ==
  data: y output; x input
function y  = fcn(x)
y=zeros(25,5);

for i=1:5
    for j=1:5
        for k=1:5
            y(5*(k-1)+i,j)=x(i,j,k);
        end
    end
end


end

== matlab function section_6_2_second_group/FUZZY3/3D-2D2 ==
  data: y output; x input
function y  = fcn(x)
y=zeros(25,5);

for i=1:5
    for j=1:5
        for k=1:5
            y(5*(k-1)+i,j)=x(i,j,k);
        end
    end
end


end

== matlab function section_6_2_second_group/FUZZY3/3D-2D3 ==
  data: y output; x input
function y  = fcn(x)
y=zeros(25,5);

for i=1:5
    for j=1:5
        for k=1:5
            y(5*(k-1)+i,j)=x(i,j,k);
        end
    end
end


end

== matlab function section_6_2_second_group/FUZZY3/3D-2D4 ==
  data: y output; x input
function y  = fcn(x)
y=zeros(25,5);

for i=1:5
    for j=1:5
        for k=1:5
            y(5*(k-1)+i,j)=x(i,j,k);
        end
    end
end


end

== matlab function section_6_2_second_group/FUZZY3/3D-2D5 ==
  data: y output; x input
function y  = fcn(x)
y=zeros(25,5);

for i=1:5
    for j=1:5
        for k=1:5
            y(5*(k-1)+i,j)=x(i,j,k);
        end
    end
end


end

== matlab function section_6_2_second_group/FUZZY3/3D-2D6 ==
  data: y output; x input
function y  = fcn(x)
y=zeros(25,5);

for i=1:5
    for j=1:5
        for k=1:5
            y(5*(k-1)+i,j)=x(i,j,k);
        end
    end
end


end

== matlab function section_6_2_second_group/FUZZY3/3D-2D7 ==
  data: y output; x input
function y  = fcn(x)
y=zeros(25,5);

for i=1:5
    for j=1:5
        for k=1:5
            y(5*(k-1)+i,j)=x(i,j,k);
        end
    end
end


end

== matlab function section_6_2_second_group/FUZZY3/3D-2D8 ==
  data: y output; x input
function y  = fcn(x)
y=zeros(25,5);

for i=1:5
    for j=1:5
        for k=1:5
            y(5*(k-1)+i,j)=x(i,j,k);
        end
    end
end


end

== matlab function section_6_2_second_group/FUZZY3/3D-2D9 ==
  data: y output; x input
function y  = fcn(x)
y=zeros(25,5);

for i=1:5
    for j=1:5
        for k=1:5
            y(5*(k-1)+i,j)=x(i,j,k);
        end
    end
end


end

== matlab function section_6_2_second_group/FUZZY3/fuzzy_adaptive_law1 ==
  data: wdot output; x1 input; x2 input; x3 input; zz input; w input
function wdot   = fcn(x1,x2,x3,zz,w)
delta=0.01;
ux1=zeros(5,1);
ux2=zeros(5,1);
ux3=zeros(5,1);
%%x1 5条模糊规则

z=zeros(5,6);
for j=1:5
    z(j,1)=-2+j-delta;
end
for j=6:10
    z(j-5,2)=-2+(j-5)-delta;
end
for j=11:15
    z(j-10,3)=-2+(j-10)-delta;
end

h1=1;%%规则间距
if x1<=-2-delta
    ux1(1,1)=1;
end

if x1>=-2-delta&&x1<=-1-delta
    ux1(1,1)=0.5*sin(pi*(x1-(-2-delta))/h1+0.5*pi)+0.5;
end

if x1>=-2-delta&&x1<=0-delta
    ux1(2,1)=0.5*sin(pi*(x1-(-1-delta))/h1+0.5*pi)+0.5;
end

if x1>=-1-delta&&x1<=1-delta
    ux1(3,1)=0.5*sin(pi*(x1-(0-delta))/h1+0.5*pi)+0.5;
end

if x1>=0-delta&&x1<=2-delta
    ux1(4,1)=0.5*sin(pi*(x1-(1-delta))/h1+0.5*pi)+0.5;
end

if x1>=1-delta&&x1<=2-delta
    ux1(5,1)=0.5*sin(pi*(x1-(2-delta))/h1+0.5*pi)+0.5;
end

if x1>2-delta
    ux1(5,1)=1;
end


h2=1;%%规则间距
if x2<=-2-delta
    ux2(1,1)=1;
end

if x2>=-2-delta&&x2<=-1-delta
    ux2(1,1)=0.5*sin(pi*(x2-(-2-delta))/h2+0.5*pi)+0.5;
end

if x2>=-2-delta&&x2<=0-delta
    ux2(2,1)=0.5*sin(pi*(x2-(-1-delta))/h2+0.5*pi)+0.5;
end

if x2>=-1-delta&&x2<=1-delta
    ux2(3,1)=0.5*sin(pi*(x2-(0-delta))/h2+0.5*pi)+0.5;
end

if x2>=0-delta&&x2<=2-delta
    ux2(4,1)=0.5*sin(pi*(x2-(1-delta))/h2+0.5*pi)+0.5;
end

if x2>=1-delta&&x2<=2-delta
    ux2(5,1)=0.5*sin(pi*(x2-(2-delta))/h2+0.5*pi)+0.5;
end

if x2>2-delta
    ux2(5,1)=1;
end

h3=1;%%规则间距
if x3<=-2-delta
    ux3(1,1)=1;
end

if x3>=-2-delta&&x3<=-1-delta
    ux3(1,1)=0.5*sin(pi*(x3-(-2-delta))/h3+0.5*pi)+0.5;
end

if x3>=-2-delta&&x3<=0-delta
    ux3(2,1)=0.5*sin(pi*(x3-(-1-delta))/h3+0.5*pi)+0.5;
end

if x3>=-1-delta&&x3<=1-delta
    ux3(3,1)=0.5*sin(pi*(x3-(0-delta))/h3+0.5*pi)+0.5;
end

if x3>=0-delta&&x3<=2-delta
    ux3(4,1)=0.5*sin(pi*(x3-(1-delta))/h3+0.5*pi)+0.5;
end

if x3>=1-delta&&x3<=2-delta
    ux3(5,1)=0.5*sin(pi*(x3-(2-delta))/h3+0.5*pi)+0.5;
end

if x3>2-delta
    ux3(5,1)=1;
end


%中心平均解模糊
Basic=0;
for i1=1:5
    for i2=1:5
        for i3=1:5
            Basic=Basic+ux1(i1,1)*ux2(i2,1)*ux3(i3,1);  
        end
    end
end

beta=zeros(5,5,5);
for i1=1:5
    for i2=1:5
        for i3=1:5
            beta(i1,i2,i3)=ux1(i1,1)*ux2(i2,1)*ux3(i3,1)/Basic;
        end
    end
end

wdot=zeros(5,5,5);
for i1=1:5
    for i2=1:5
        for i3=1:5
            wdot(i1,i2,i3)=w*beta(i1,i2,i3)*zz*z(i3,1);
        end
    end
end

end

== matlab function section_6_2_second_group/FUZZY3/fuzzy_adaptive_law2 ==
  data: wdot output; x1 input; x2 input; x3 input; zz input; w input
function wdot   = fcn(x1,x2,x3,zz,w)
delta=0.01;
ux1=zeros(5,1);
ux2=zeros(5,1);
ux3=zeros(5,1);
%%x1 5条模糊规则

z=zeros(5,6);
for j=1:5
    z(j,1)=-2+j-delta;
end
for j=6:10
    z(j-5,2)=-2+(j-5)-delta;
end
for j=11:15
    z(j-10,3)=-2+(j-10)-delta;
end

h1=1;%%规则间距
if x1<=-2-delta
    ux1(1,1)=1;
end

if x1>=-2-delta&&x1<=-1-delta
    ux1(1,1)=0.5*sin(pi*(x1-(-2-delta))/h1+0.5*pi)+0.5;
end

if x1>=-2-delta&&x1<=0-delta
    ux1(2,1)=0.5*sin(pi*(x1-(-1-delta))/h1+0.5*pi)+0.5;
end

if x1>=-1-delta&&x1<=1-delta
    ux1(3,1)=0.5*sin(pi*(x1-(0-delta))/h1+0.5*pi)+0.5;
end

if x1>=0-delta&&x1<=2-delta
    ux1(4,1)=0.5*sin(pi*(x1-(1-delta))/h1+0.5*pi)+0.5;
end

if x1>=1-delta&&x1<=2-delta
    ux1(5,1)=0.5*sin(pi*(x1-(2-delta))/h1+0.5*pi)+0.5;
end

if x1>2-delta
    ux1(5,1)=1;
end


h2=1;%%规则间距
if x2<=-2-delta
    ux2(1,1)=1;
end

if x2>=-2-delta&&x2<=-1-delta
    ux2(1,1)=0.5*sin(pi*(x2-(-2-delta))/h2+0.5*pi)+0.5;
end

if x2>=-2-delta&&x2<=0-delta
    ux2(2,1)=0.5*sin(pi*(x2-(-1-delta))/h2+0.5*pi)+0.5;
end

if x2>=-1-delta&&x2<=1-delta
    ux2(3,1)=0.5*sin(pi*(x2-(0-delta))/h2+0.5*pi)+0.5;
end

if x2>=0-delta&&x2<=2-delta
    ux2(4,1)=0.5*sin(pi*(x2-(1-delta))/h2+0.5*pi)+0.5;
end

if x2>=1-delta&&x2<=2-delta
    ux2(5,1)=0.5*sin(pi*(x2-(2-delta))/h2+0.5*pi)+0.5;
end

if x2>2-delta
    ux2(5,1)=1;
end

h3=1;%%规则间距
if x3<=-2-delta
    ux3(1,1)=1;
end

if x3>=-2-delta&&x3<=-1-delta
    ux3(1,1)=0.5*sin(pi*(x3-(-2-delta))/h3+0.5*pi)+0.5;
end

if x3>=-2-delta&&x3<=0-delta
    ux3(2,1)=0.5*sin(pi*(x3-(-1-delta))/h3+0.5*pi)+0.5;
end

if x3>=-1-delta&&x3<=1-delta
    ux3(3,1)=0.5*sin(pi*(x3-(0-delta))/h3+0.5*pi)+0.5;
end

if x3>=0-delta&&x3<=2-delta
    ux3(4,1)=0.5*sin(pi*(x3-(1-delta))/h3+0.5*pi)+0.5;
end

if x3>=1-delta&&x3<=2-delta
    ux3(5,1)=0.5*sin(pi*(x3-(2-delta))/h3+0.5*pi)+0.5;
end

if x3>2-delta
    ux3(5,1)=1;
end


%中心平均解模糊
Basic=0;
for i1=1:5
    for i2=1:5
        for i3=1:5
            Basic=Basic+ux1(i1,1)*ux2(i2,1)*ux3(i3,1);  
        end
    end
end

beta=zeros(5,5,5);
for i1=1:5
    for i2=1:5
        for i3=1:5
            beta(i1,i2,i3)=ux1(i1,1)*ux2(i2,1)*ux3(i3,1)/Basic;
        end
    end
end

wdot=zeros(5,5,5);
for i1=1:5
    for i2=1:5
        for i3=1:5
            wdot(i1,i2,i3)=w*beta(i1,i2,i3)*zz*z(i3,1);
        end
    end
end

end
